simulink model "rtlsdr_fm_pll_stereo_demod"  (R2014b)
settings: Solver=ode45  StartTime=0.0  StopTime=30  RelTol=1e-3
PreLoadFcn:
  | %%%%%%%%%%%%%%%%%%%%%%%%%%%%%%%%%%%%%%%%%%%%%%%%%%%%%%%%%%%%%%%%%%%%%%%%%%%
  | % check to see if Simulink library folder is missing from the MATLAB path %
  | %%%%%%%%%%%%%%%%%%%%%%%%%%%%%%%%%%%%%%%%%%%%%%%%%%%%%%%%%%%%%%%%%%%%%%%%%%%
  | if isempty(strfind(path, 'rtlsdr_book_library'))
  | 
  |     % create error window
  |     fig_error = figure(...
  |         'Name', 'Error: RTL-SDR Book Library',...
  |         'Toolbar','none',...
  |         'MenuBar','none',...
  |         'NumberTitle','off',...
  |         'Resize','off',...
  |         'WindowStyle','modal');
  |     fig_error.Position(3) = 600;
  |     fig_error.Position(4) = 150;
  |     fig_axes = axes(...
  |         'Parent',fig_error,...
  |         'Position',[0,0,1,1],...
  |         'visible','off');
  |     % error message
  |     t_title = text(.05,.8,...
  |         'MISSING DIRECTORIES',...
  |         'FontSize',11.5);
  |     t_body = text(.075,.6,...
  |         [{'Simulink cannot find the  \it{<root>}\rm / \it{rtlsdr\_book\_library}\rm  folder in the \it{MATLAB Path}\rm.'},...
  |         {'Please set the MATLAB path following the instructions given in Exercise 2.4.'}],...
  |         'FontSize',10.5);
  |     % buttons
  |     btn_path = uicontrol(...
  |         'Parent',fig_error,...
  |         'String','Set Path Now',...
  |         'FontSize',10,...
  |         'Callback', 'pathtool; close(fig_error);',...
  |         'Position', [fig_error.Position(3)/2-210, 30, 200, 30]);
  |     btn_abort = uicontrol(...
  |         'Parent',fig_error,...
  |         'String','No thanks',...
  |         'FontSize',10,...
  |         'Callback', 'close(fig_error); abort=1;',...
  |         'Position', [fig_error.Position(3)/2+10, 30, 200, 30]);
  | 
  |     % pause to allow user to interact with error box
  |     uiwait(fig_error);
  | 
  |     % abort simulation
  |     try
  |         if abort==1
  |             set_param(gcs, 'SimulationCommand', 'stop');
  |         end
  |     end
  | 
  |     % if user has set path, allow diagram to be updated
  |     if ~exist('abort','var')
  |         % create error window
  |         fig_update = figure(...
  |             'Name', 'Update Diagram',...
  |             'Toolbar','none',...
  |             'MenuBar','none',...
  |             'NumberTitle','off',...
  |             'Resize','off');
  |         fig_update.Position(3) = 400;
  |         fig_update.Position(4) = 120;
  |         fig_axes = axes(...
  |             'Parent',fig_update,...
  |             'Position',[0,0,1,1],...
  |             'visible','off');
  |         % instruction message
  |         t_body = text(.075,.7,...
  |             'Once you have set the path, update the block diagram',...
  |             'FontSize',10.5);
  |         % button
  |         btn_update = uicontrol(...
  |             'Parent',fig_update,...
  |             'String','Update Block Diagram',...
  |             'FontSize',10,...
  |             'Callback', 'set_param(gcs,''SimulationCommand'',''update''); close(gcf)',...
  |             'Position', [fig_update.Position(3)/2-100, 30, 200, 30]);
  |     end
  | 
  |     % clear error components
  |     clear('fig_error','fig_update','fig_axes','t_title','t_body','btn_path','btn_abort','btn_update','abort');
  | 
  | end
  | %%%%%%%%%%%%%%%%%%%%%%%%%%%%%%%%%%%%%%%%%%%%%%%%%%%%%%%%%%%%%%%%%%%%%%%%%%%
undefined symbols (not defined in the file or in its folder): Bn, d, fs, Ko, Kp, startfcn_spectrum_analyzer
libraries: rtlsdr_book_library x5, dspmlti4 x3, commrfcorlib x1, dspvision x1
CloseFcn:
  | closefcn_model
Description:
  | Software, Simulation Examples and Design Exercises Licence Agreement
  | 
  | This license agreement refers to the simulation examples, design exercises and files,
  | and associated software MATLAB and Simulink resources that accompany the book:
  | 
  |      Title: Software Defined Radio using MATLAB & Simulink and the RTL-SDR
  |      Published by Strathclyde Academic Media, 2015
  |      Authored by Robert W. Stewart, Kenneth W. Barlee, Dale S.W. Atkinson,
  |      and Louise H. Crockett
  | 
  | and made available as a download from, www.desktopSDR.com or variously acquired
  | by other means such as via USB storage, cloud storage, disk or any other electronic
  | or optical or magnetic storage mechanism. These files and associated software may
  | be used subject to the terms of agreement of the conditions below:
  | 
  |     Copyright © 2015 Robert W. Stewart, Kenneth W. Barlee, Dale S.W. Atkinson,
  |     and Louise H. Crockett
  |     All rights reserved.
  | 
  | Redistribution and use in source and binary forms, with or without modification, are
  | permitted provided that the following conditions are met:
  | 
  |    1.  Redistributions of source code must retain the above copyright notice, this list of
  |         conditions and the following disclaimer.
  | 
  |    2.  Redistributions in binary form must reproduce the above copyright notice, this
  |         list of conditions and the following disclaimer in the documentation and/or other
  |         materials provided with the distribution.
  | 
  |    3.  Neither the name of the copyright holder nor the names of its contributors may
  |         be used to endorse or promote products derived from this software without
  |         specific prior written permission.
  | 
  |    4.  In all cases, the software is, and all modifications and derivatives of the
  |         software shall be, licensed to you solely for use in conjunction with The
  |         MathWorks, Inc. products and service offerings.
  | 
  | THIS SOFTWARE IS PROVIDED BY THE COPYRIGHT HOLDERS AND CONTRIBUTORS
  | "AS IS" AND ANY EXPRESS OR IMPLIED WARRANTIES, INCLUDING, BUT NOT LIMITED
  | TO, THE IMPLIED WARRANTIES OF MERCHANTABILITY AND FITNESS FOR A
  | PARTICULAR PURPOSE ARE DISCLAIMED. IN NO EVENT SHALL THE COPYRIGHT
  | HOLDER OR CONTRIBUTORS BE LIABLE FOR ANY DIRECT, INDIRECT, INCIDENTAL,
  | SPECIAL, EXEMPLARY, OR CONSEQUENTIAL DAMAGES (INCLUDING, BUT NOT
  | LIMITED TO, PROCUREMENT OF SUBSTITUTE GOODS OR SERVICES; LOSS OF USE,
  | DATA, OR PROFITS; OR BUSINESS INTERRUPTION) HOWEVER CAUSED AND ON ANY
  | THEORY OF LIABILITY, WHETHER IN CONTRACT, STRICT LIABILITY, OR TORT
  | (INCLUDING NEGLIGENCE OR OTHERWISE) ARISING IN ANY WAY OUT OF THE USE
  | OF THIS SOFTWARE, EVEN IF ADVISED OF THE POSSIBILITY OF SUCH DAMAGE.
  | 
  | 
  | Audio Tracks used in Simulations Examples and Design Exercises
  | 
  | The music and vocal files used within the Examples files and software within the book
  | were variously written, arranged, performed, recorded and produced by Garrey Rice,
  | Adam Struth, Jamie Struth, Iain Thistlethwaite and also Marshall Craigmyle who
  | collectively, and individually where appropriate, assert and retain all of their copyright,
  | performance and artistic rights. Permission to use and reproduce this music is
  | granted for all purposes associated with MATLAB and Simulink software and the
  | simulation examples and design exercises files that accompany this book. Requests to
  | use the music for any other purpose should be directed to: info@desktopSDR.com.
  | For information on music track names, full credits, and links to the musicians please
  | refer to www.desktopSDR.com/more/audio.
settings Model: SimulationMode=accelerator  Creator=desktopSDR Team  LastModifiedBy=desktopSDR Team
settings DataIOCC: LimitDataPoints=off  SaveOutput=off  SignalLogging=off  SaveTime=off

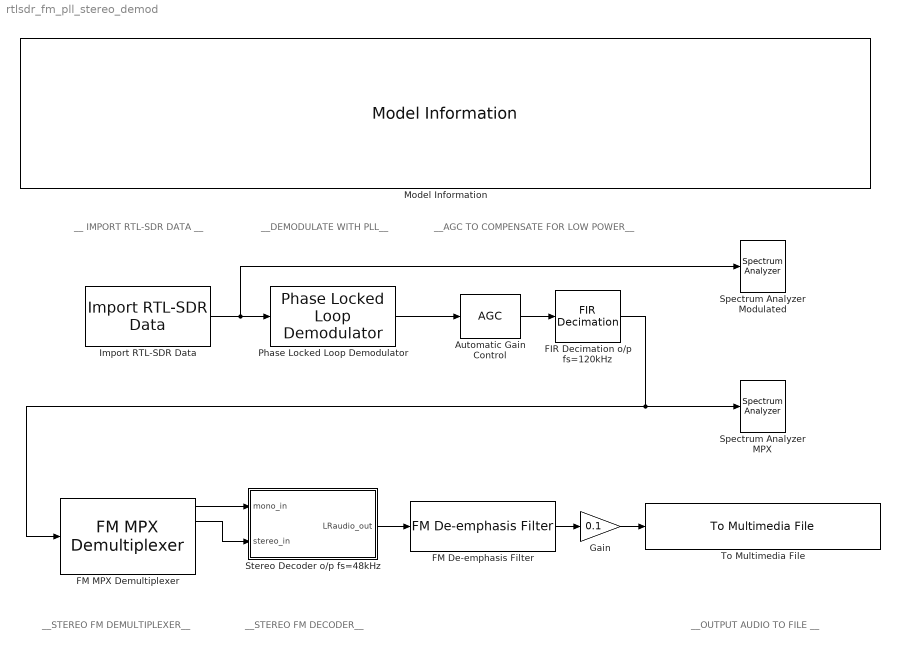
== system rtlsdr_fm_pll_stereo_demod ==
  note: __ IMPORT RTL-SDR DATA __
  note: __OUTPUT AUDIO TO FILE __
  note: __DEMODULATE WITH PLL__
  note: __STEREO FM DEMULTIPLEXER__
  note: __STEREO FM DECODER__
  note: __AGC TO COMPENSATE FOR LOW POWER__
  Automatic Gain Control : commrfcorlib/AGC  SimulateUsing=Code generation  DetectorMethod=Rectifier  LoopMethod=Linear  UpdatePeriod=4096  StepSize=0.1  MaximumGain=20  GainOutputPort=off
  FIR Decimation o/p fs=120kHz : dspmlti4/FIR Decimation  h=firpm(50, [0 60e3 120e3 (1.2e6/2)]/(1.2e6/2), [1 1 0 0], [1 1],20)  D=10  filtStruct=Direct form  framing=Allow multirate processing  inputOffset=0  outputBufInitCond=0  InputProcessing=Columns as channels (frame based)  firstCoeffDataTypeStr=Inherit: Same word length as input  firstCoeffLastDataTypeStr=Inherit: Same word length as input  firstCoeffMin=[]  firstCoeffMax=[]  outputDataTypeStr=Inherit: Same as accumulator  outputLastDataTypeStr=Inherit: Same as accumulator  outputMin=[]  outputMax=[]  roundingMode=Floor  overflowMode=off  FilterSource=Specify via dialog  FilterObject=Hm_firdecim
      settings: allowOverrides=off
  FM De-emphasis Filter : rtlsdr_book_library/FM Demod Tools/FM De-emphasis Filter  region=Europe, Asia  fs=48e3
  FM MPX Demultiplexer : rtlsdr_book_library/FM Demod Tools/FM MPX Demultiplexer  fs=120e3  fq=19e3  Kpd=3  Kphe=2  frm_size=4000
  Gain : Gain  Gain=0.1
  Import RTL-SDR Data : rtlsdr_book_library/Additional Tools/Import RTL-SDR Data  filename=rec_data\wfm_stereo_150kHzoffset.mat  frm_size=4096  data_type=single
  Model Information : rtlsdr_book_library/Additional Tools/Model Information/Model Information
  Phase Locked Loop Demodulator : rtlsdr_book_library/Sync Tools for Analogue Comms/Phase Locked Loop Demodulator  filter_type=Type 2  K1_param=(4*d*Bn*1/fs)/(Ko*Kp*(d+1/(4*d)))  K2_param=(4*(Bn*1/fs)^2)/(Ko*Kp*(d+1/4*d)^2)  fs=1.2e6  fq=150e3  Bn=37.5e3  d=1  frm_size=4096
  Spectrum Analyzer MPX : SpectrumAnalyzer  StartFcn=startfcn_spectrum_analyzer;
  Spectrum Analyzer Modulated : SpectrumAnalyzer  StartFcn=startfcn_spectrum_analyzer;
  Stereo Decoder o/p fs=48kHz : Subsystem
  To Multimedia File : dspvision/To Multimedia File  outputFilename=rtlsdr_fm_pll_stereo_demod.wav  streamSelection=Audio only  videoCompressor=None (uncompressed)  audioCompressor=None (uncompressed)  imagePorts=Separate color signals  fileType=WAV  audioDatatype=16-bit integer  fourcc=RGB  videoQuality=75  mj2000CompFactor=10
  wires:
  Phase Locked Loop Demodulator/2 -> Automatic Gain Control/1
  Automatic Gain Control/1 -> FIR Decimation o/p fs=120kHz/1
  FM De-emphasis Filter/1 -> Gain/1
  FIR Decimation o/p fs=120kHz/1 -> FM MPX Demultiplexer/1, Spectrum Analyzer MPX/1
  Stereo Decoder o/p fs=48kHz/1(LRaudio_out) -> FM De-emphasis Filter/1
  FM MPX Demultiplexer/1 -> Stereo Decoder o/p fs=48kHz/1(mono_in)
  FM MPX Demultiplexer/2 -> Stereo Decoder o/p fs=48kHz/2(stereo_in)
  Gain/1 -> To Multimedia File/1
  Import RTL-SDR Data/1 -> Phase Locked Loop Demodulator/1, Spectrum Analyzer Modulated/1

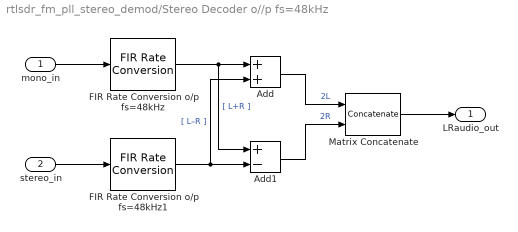
== system rtlsdr_fm_pll_stereo_demod/Stereo Decoder o//p fs=48kHz ==
  mono_in : Inport
  stereo_in : Inport  Port=2
  Add : Sum
  Add1 : Sum  Inputs=+-
  FIR Rate Conversion o/p fs=48kHz : dspmlti4/FIR Rate Conversion  L=2  h=firpm(100, [0 15e3 20e3 240e3/2]/(240e3/2), [1 1 0 0], [1 1],20)  M=5  firstCoeffDataTypeStr=Inherit: Same word length as input  firstCoeffLastDataTypeStr=Inherit: Same word length as input  firstCoeffMin=[]  firstCoeffMax=[]  outputDataTypeStr=Inherit: Same as accumulator  outputLastDataTypeStr=Inherit: Same as accumulator  outputMin=[]  outputMax=[]  roundingMode=Floor  overflowMode=off  FilterSource=Specify via dialog  FilterObject=Hm_firsrc
  FIR Rate Conversion o/p fs=48kHz1 : dspmlti4/FIR Rate Conversion  L=2  h=firpm(100, [0 15e3 20e3 240e3/2]/(240e3/2), [1 1 0 0], [1 1],20)  M=5  firstCoeffDataTypeStr=Inherit: Same word length as input  firstCoeffLastDataTypeStr=Inherit: Same word length as input  firstCoeffMin=[]  firstCoeffMax=[]  outputDataTypeStr=Inherit: Same as accumulator  outputLastDataTypeStr=Inherit: Same as accumulator  outputMin=[]  outputMax=[]  roundingMode=Floor  overflowMode=off  FilterSource=Specify via dialog  FilterObject=Hm_firsrc
  Matrix Concatenate : Concatenate  Mode=Multidimensional array  ConcatenateDimension=2
  LRaudio_out : Outport
  wires:
  Add1/1 -> Matrix Concatenate/2  "2R"
  FIR Rate Conversion o/p fs=48kHz/1 -> Add/1, Add1/1  "[ L+R ]"
  mono_in/1 -> FIR Rate Conversion o/p fs=48kHz/1
  stereo_in/1 -> FIR Rate Conversion o/p fs=48kHz1/1
  Add/1 -> Matrix Concatenate/1  "2L"
  FIR Rate Conversion o/p fs=48kHz1/1 -> Add1/2, Add/2  "[ L–R ]"
  Matrix Concatenate/1 -> LRaudio_out/1
